simulink model "SimulinkModel"  (Simulink 8.3)
settings: Solver=ode45  StartTime=0.0  StopTime=20  RelTol=1e-3
settings Model: Creator=Administrator  LastModifiedBy=JimmyChen
settings DataIOCC: SignalLoggingSaveFormat=Dataset
settings DebuggingCC: UnderspecifiedInitializationDetection=Simplified  StateNameClashWarn=none
settings GRTTargetCC: CombineOutputUpdateFcns=on  GRTInterface=off

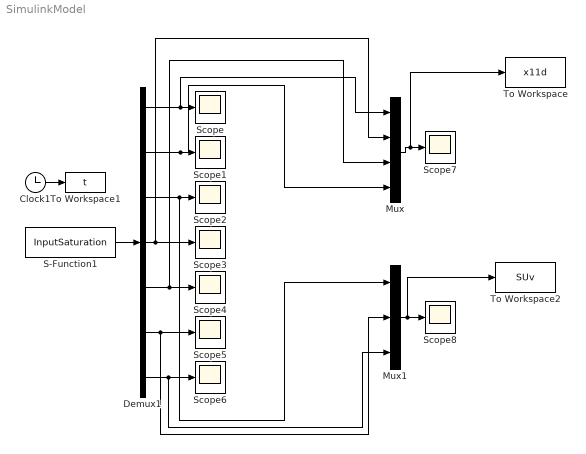
== system SimulinkModel ==
  Clock1 : Clock
  Demux1 : Demux  Outputs=7
  Mux : Mux
  Mux1 : Mux  Inputs=3
  S-Function1 : S-Function  FunctionName=InputSaturation  EnableBusSupport=off
  Scope{,1..8} (9 alike) : Scope
      Scope2 settings: SaveName=ScopeData2
      Scope3 settings: SaveName=ScopeData3
      Scope4 settings: SaveName=ScopeData4
      Scope5 settings: SaveName=ScopeData5
      Scope6 settings: SaveName=ScopeData6
      Scope7 settings: SaveName=ScopeData7
      Scope8 settings: SaveName=ScopeData8
  To Workspace : ToWorkspace  VariableName=x11d  SaveFormat=Timeseries  SampleTime=-1
  To Workspace1 : ToWorkspace  VariableName=t  SaveFormat=Timeseries  SampleTime=-1
  To Workspace2 : ToWorkspace  VariableName=SUv  SaveFormat=Timeseries  SampleTime=-1
  wires:
  S-Function1/1 -> Demux1/1
  Clock1/1 -> To Workspace1/1
  Demux1/1 -> Mux/1, Scope/1
  Demux1/2 -> Mux/4, Scope1/1
  Demux1/3 -> Mux1/1, Scope2/1
  Demux1/4 -> Mux/2, Scope3/1
  Demux1/5 -> Mux/3, Scope4/1
  Demux1/6 -> Mux1/2, Scope5/1
  Demux1/7 -> Mux1/3, Scope6/1
  Mux/1 -> To Workspace/1, Scope7/1
  Mux1/1 -> To Workspace2/1, Scope8/1
